simulink model "MRAC_controller"  (R2021b)
settings: Solver=ode113  StartTime=0.0  StopTime=10  RelTol=1e-3
InitFcn:
  | addpath('generated');
  | cst = cellulo_constants();
  | 
  | Td_sens = 0.02;
  | T_ctrl = 0.02;
  | c = cst.c;
  | c_v=cst.c_v;
  | c_F=cst.c_F;
  | c_U = cst.c_U;
  | m = cst.m;
  | d=cst.d;
  | M=mass();
  | 
  | constants = [cst.d;
  |                    cst.c;
  |                    cst.c_F;
  |                    cst.c_U;
  |                    cst.c_v;
  |                    cst.I_drive;
  |                    cst.I_wheel;
  |                    cst.Iz;
  |                    cst.r_mag;
  |                    cst.r_wheel];
  | 
  | rng('default');
  | r = rand(size(constants))/2-0.2;
  | constants = constants + r.*constants;
model workspace (MAT data in the model file):
  Td = 0.1
settings Model: Creator=Hadrien  LastModifiedBy=Hadrien
settings SolverCC: AlgebraicLoopSolver=TrustRegion
settings DebuggingCC: SFMachineParentedDataDiag=warning

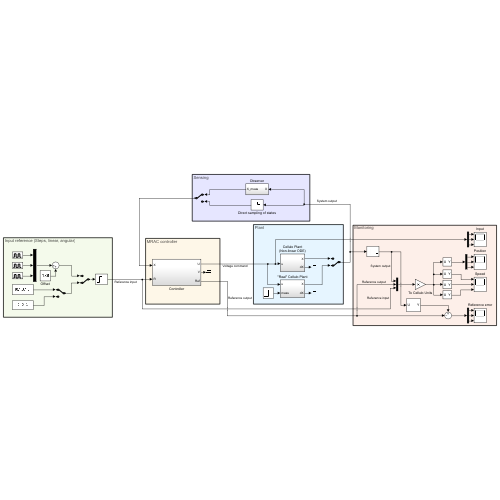
[thumbnail: Simulink's stored preview of the top-level diagram]
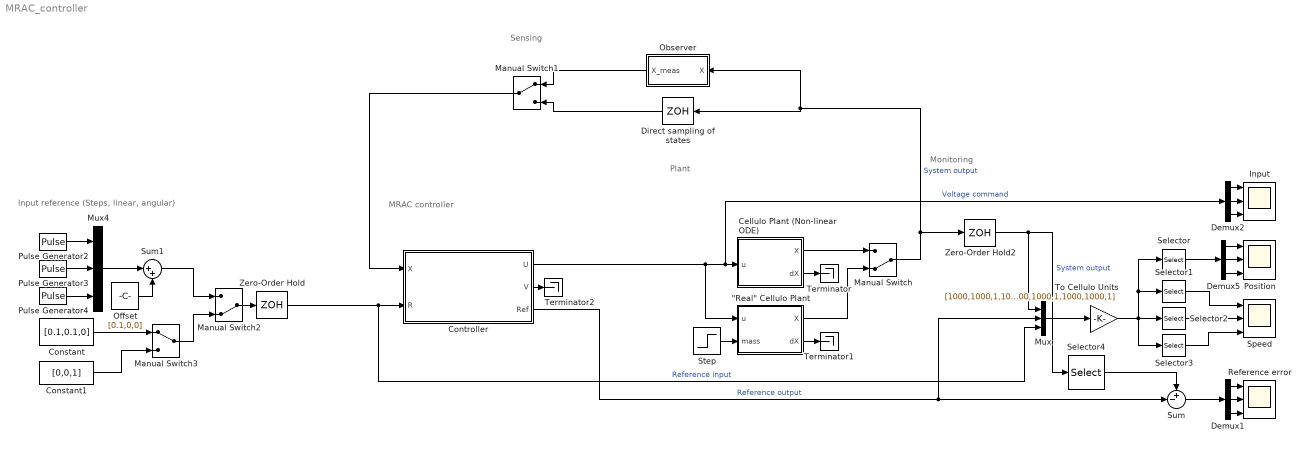
== system MRAC_controller ==
  note: Monitoring
  note: MRAC controller
  note: Plant
  note: Sensing
  note: Input reference (Steps, linear, angular)
  "\"Real\" Cellulo Plant" : Subsystem
  Cellulo Plant (Non-linear ODE) : Subsystem
  Constant : Constant  Value=[0.1,0.1,0]
  Constant1 : Constant  Value=[0,0,1]
  Controller : Subsystem
  Demux1 : Demux  Outputs=3
  Demux2 : Demux  Outputs=3
  Demux5 : Demux  Outputs=3
  Direct sampling of states : ZeroOrderHold  SampleTime=Td_sens
  Input : Scope  NumInputPorts=3
  Manual Switch : ManualSwitch  CurrentSetting=0
  Manual Switch1 : ManualSwitch
  Manual Switch2 : ManualSwitch  CurrentSetting=0
  Manual Switch3 : ManualSwitch
  Mux : Mux  Inputs=3
  Mux4 : Mux  Inputs=3
  Observer : Subsystem
  Offset : Constant  Value=[0.1,0,0]
  Position : Scope  NumInputPorts=3
  Pulse Generator2 : DiscretePulseGenerator  PulseType=Time based  Amplitude=0.1  Period=9  PulseWidth=50  SampleTime=T_ctrl
  Pulse Generator3 : DiscretePulseGenerator  PulseType=Time based  Amplitude=0.1  Period=10  PulseWidth=50  PhaseDelay=2  SampleTime=T_ctrl
  Pulse Generator4 : DiscretePulseGenerator  PulseType=Time based  Period=8  PulseWidth=50  PhaseDelay=1  SampleTime=T_ctrl
  Reference error : Scope  NumInputPorts=3
  Selector : Selector  InputPortWidth=12  IndexOptions=Index vector (dialog)  Indices=[1 2 3]  OutputSizes=1
  Selector1 : Selector  InputPortWidth=12  IndexOptions=Index vector (dialog)  Indices=[4 7 10]  OutputSizes=1
  Selector2 : Selector  InputPortWidth=12  IndexOptions=Index vector (dialog)  Indices=[5 8 11]  OutputSizes=1
  Selector3 : Selector  InputPortWidth=12  IndexOptions=Index vector (dialog)  Indices=[6 9 12]  OutputSizes=1
  Selector4 : Selector  InputPortWidth=6  IndexOptions=Index vector (dialog)  Indices=[4 5 6]  OutputSizes=1
  Speed : Scope  NumInputPorts=3
  Step : Step  Time=0  Before=m  After=10*m  SampleTime=0
  Sum : Sum  Inputs=+-|
  Sum1 : Sum  Inputs=|++
  Terminator : Terminator
  Terminator1 : Terminator
  Terminator2 : Terminator
  To Cellulo Units : Gain  Gain=[1000,1000,1,1000,1000,1,1000,1000,1,1000,1000,1]
  Zero-Order Hold : ZeroOrderHold  SampleTime=T_ctrl
  Zero-Order Hold2 : ZeroOrderHold  SampleTime=T_ctrl
  wires:
  Cellulo Plant (Non-linear ODE)/2(dX) -> Terminator/1
  "\"Real\" Cellulo Plant"/2(dX) -> Terminator1/1
  "\"Real\" Cellulo Plant"/1(X) -> Manual Switch/2
  Cellulo Plant (Non-linear ODE)/1(X) -> Manual Switch/1
  Manual Switch/1 -> Observer/1(X), Direct sampling of states/1, Zero-Order Hold2/1  "System output"
  Observer/1(X_meas) -> Manual Switch1/1
  Direct sampling of states/1 -> Manual Switch1/2
  Controller/1(U) -> Demux2/1, Cellulo Plant (Non-linear ODE)/1(u), "\"Real\" Cellulo Plant"/1(u)  "Voltage command"
  Manual Switch1/1 -> Controller/1(X)
  Step/1 -> "\"Real\" Cellulo Plant"/2(mass)
  Pulse Generator2/1 -> Mux4/1
  Pulse Generator4/1 -> Mux4/3
  Pulse Generator3/1 -> Mux4/2
  Mux/1 -> To Cellulo Units/1
  Selector/1 -> Demux5/1
  Demux5/2 -> Position/2
  Demux5/1 -> Position/1
  Demux5/3 -> Position/3
  Selector1/1 -> Speed/1
  Selector2/1 -> Speed/2
  Selector3/1 -> Speed/3
  To Cellulo Units/1 -> Selector1/1, Selector/1, Selector3/1, Selector2/1
  Zero-Order Hold2/1 -> Selector4/1, Mux/1  "System output"
  Controller/3(Ref) -> Mux/2, Sum/2  "Reference output"
  Demux2/1 -> Input/1
  Demux2/2 -> Input/2
  Demux2/3 -> Input/3
  Controller/2(V) -> Terminator2/1
  Demux1/3 -> Reference error/3
  Demux1/1 -> Reference error/1
  Demux1/2 -> Reference error/2
  Manual Switch2/1 -> Zero-Order Hold/1
  Manual Switch3/1 -> Manual Switch2/2
  Constant/1 -> Manual Switch3/1
  Constant1/1 -> Manual Switch3/2
  Mux4/1 -> Sum1/1
  Sum1/1 -> Manual Switch2/1
  Offset/1 -> Sum1/2
  Zero-Order Hold/1 -> Mux/3, Controller/2(R)  "Reference input"
  Sum/1 -> Demux1/1
  Selector4/1 -> Sum/1

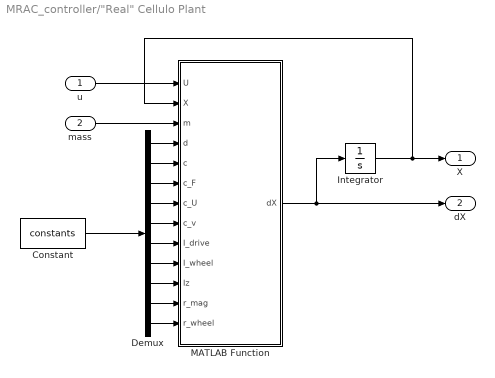
== system MRAC_controller/"Real" Cellulo Plant ==
  u : Inport  PortDimensions=3
  mass : Inport  Port=2
  Constant : Constant  Value=constants
  Demux : Demux  Outputs=10
  Integrator : Integrator
  MATLAB Function : MATLAB Function  TreatAsAtomicUnit=on
  X : Outport  PortDimensions=6
  dX : Outport  Port=2  PortDimensions=6
  wires:
  Integrator/1 -> X/1, MATLAB Function/2(X)
  u/1 -> MATLAB Function/1(U)
  MATLAB Function/1(dX) -> Integrator/1, dX/1
  Demux/1 -> MATLAB Function/4(d)
  Demux/2 -> MATLAB Function/5(c)
  Demux/3 -> MATLAB Function/6(c_F)
  Demux/4 -> MATLAB Function/7(c_U)
  Demux/5 -> MATLAB Function/8(c_v)
  Demux/6 -> MATLAB Function/9(I_drive)
  Demux/7 -> MATLAB Function/10(I_wheel)
  Demux/8 -> MATLAB Function/11(Iz)
  Demux/9 -> MATLAB Function/12(r_mag)
  Demux/10 -> MATLAB Function/13(r_wheel)
  Constant/1 -> Demux/1
  mass/1 -> MATLAB Function/3(m)

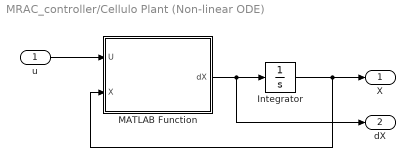
== system MRAC_controller/Cellulo Plant (Non-linear ODE) ==
  u : Inport  PortDimensions=3
  Integrator : Integrator
  MATLAB Function : MATLAB Function  TreatAsAtomicUnit=on
  X : Outport  PortDimensions=6
  dX : Outport  Port=2  PortDimensions=6
  wires:
  u/1 -> MATLAB Function/1(U)
  MATLAB Function/1(dX) -> Integrator/1, dX/1
  Integrator/1 -> MATLAB Function/2(X), X/1

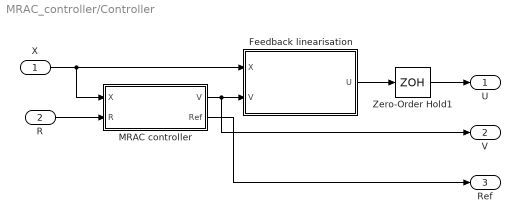
== system MRAC_controller/Controller ==
  X : Inport
  R : Inport  Port=2
  Feedback linearisation : MATLAB Function  TreatAsAtomicUnit=on
  MRAC controller : Subsystem
  Zero-Order Hold1 : ZeroOrderHold  SampleTime=-1
  U : Outport
  V : Outport  Port=2
  Ref : Outport  Port=3
  wires:
  X/1 -> Feedback linearisation/1(X), MRAC controller/1(X)
  R/1 -> MRAC controller/2(R)
  Feedback linearisation/1(U) -> Zero-Order Hold1/1
  MRAC controller/1(V) -> Feedback linearisation/2(V), V/1
  Zero-Order Hold1/1 -> U/1
  MRAC controller/2(Ref) -> Ref/1

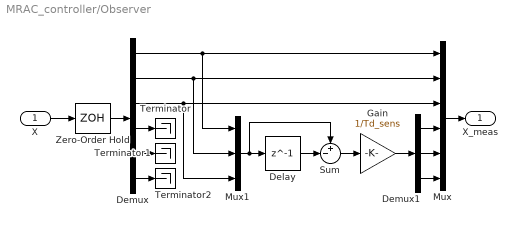
== system MRAC_controller/Observer ==
  X : Inport
  Delay : Delay  DelayLength=1  SampleTime=Td_sens
  Demux : Demux  Outputs=6
  Demux1 : Demux  Outputs=3
  Gain : Gain  Gain=1/Td_sens
  Mux : Mux  Inputs=6
  Mux1 : Mux  Inputs=3
  Sum : Sum  Inputs=+-|
  Terminator : Terminator
  Terminator1 : Terminator
  Terminator2 : Terminator
  Zero-Order Hold : ZeroOrderHold  SampleTime=Td_sens
  X_meas : Outport
  wires:
  X/1 -> Zero-Order Hold/1
  Zero-Order Hold/1 -> Demux/1
  Mux/1 -> X_meas/1
  Demux/1 -> Mux/1, Mux1/1
  Demux/2 -> Mux/2, Mux1/2
  Demux/3 -> Mux/3, Mux1/3
  Demux/4 -> Terminator/1
  Demux/5 -> Terminator1/1
  Demux/6 -> Terminator2/1
  Demux1/1 -> Mux/4
  Demux1/2 -> Mux/5
  Demux1/3 -> Mux/6
  Sum/1 -> Gain/1
  Mux1/1 -> Sum/1, Delay/1
  Delay/1 -> Sum/2
  Gain/1 -> Demux1/1

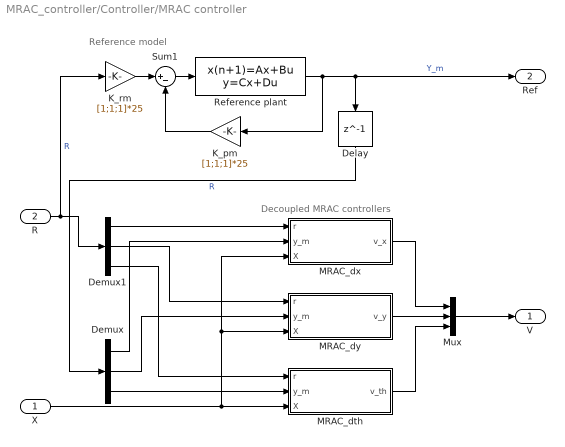
== system MRAC_controller/Controller/MRAC controller ==
  note: Decoupled MRAC controllers
  note: Reference model
  X : Inport
  R : Inport  Port=2
  Delay : Delay  DelayLength=1
  Demux : Demux  Outputs=3
  Demux1 : Demux  Outputs=3
  K_pm : Gain  Gain=[1;1;1]*25
  K_rm : Gain  Gain=[1;1;1]*25
  MRAC_dth : Subsystem
  MRAC_dx : Subsystem
  MRAC_dy : Subsystem
  Mux : Mux  Inputs=3
  Reference plant : DiscreteStateSpace  A=eye(3)  B=T_ctrl*eye(3)  C=eye(3)  D=zeros(3)  SampleTime=-1
  Sum1 : Sum  Inputs=|+-
  V : Outport
  Ref : Outport  Port=2
  wires:
  K_pm/1 -> Sum1/2
  K_rm/1 -> Sum1/1
  Sum1/1 -> Reference plant/1
  Reference plant/1 -> Ref/1, Delay/1, K_pm/1  "Y_m"
  Demux/1 -> MRAC_dx/2(y_m)
  Demux1/1 -> MRAC_dx/1(r)
  X/1 -> MRAC_dy/3(X), MRAC_dx/3(X), MRAC_dth/3(X)
  MRAC_dx/1(v_x) -> Mux/1
  Demux1/2 -> MRAC_dy/1(r)
  Demux1/3 -> MRAC_dth/1(r)
  Demux/2 -> MRAC_dy/2(y_m)
  Demux/3 -> MRAC_dth/2(y_m)
  MRAC_dy/1(v_y) -> Mux/2
  MRAC_dth/1(v_th) -> Mux/3
  Mux/1 -> V/1
  R/1 -> K_rm/1, Demux1/1  "R"
  Delay/1 -> Demux/1  "R"

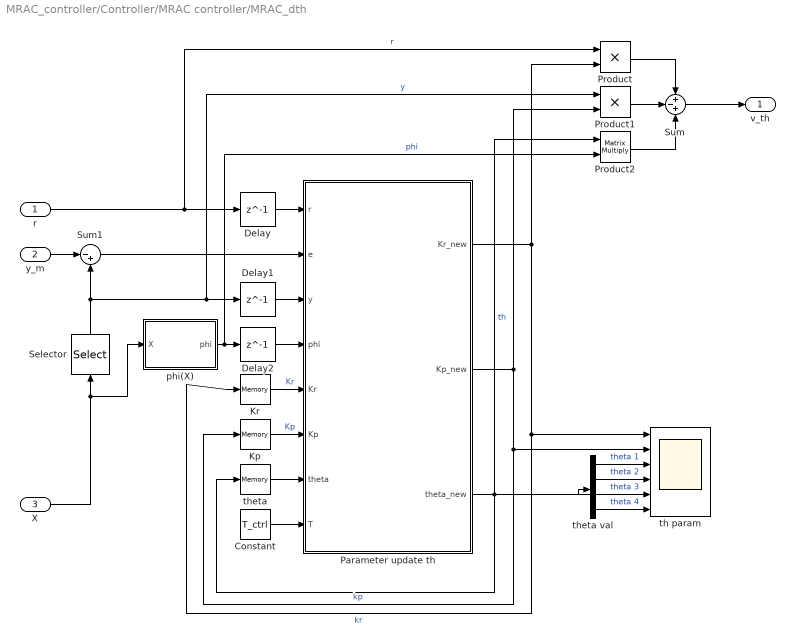
== system MRAC_controller/Controller/MRAC controller/MRAC_dth ==
  r : Inport
  y_m : Inport  Port=2
  X : Inport  Port=3
  Constant : Constant  Value=T_ctrl
  Delay : Delay  DelayLength=1
  Delay1 : Delay  DelayLength=1
  Delay2 : Delay  DelayLength=1
  Kp : Memory  InitialCondition=118  InheritSampleTime=on
  Kr : Memory  InitialCondition=119  InheritSampleTime=on
  Parameter update th : MATLAB Function  TreatAsAtomicUnit=on
  Product : Product
  Product1 : Product
  Product2 : Product  Multiplication=Matrix(*)
  Selector : Selector  InputPortWidth=6  IndexOptions=Index vector (dialog)  Indices=6  OutputSizes=1
  Sum : Sum  Inputs=+-+
  Sum1 : Sum  Inputs=|-+
  phi(X) : MATLAB Function  TreatAsAtomicUnit=on
  th param : Scope  NumInputPorts=6
  theta : Memory  InitialCondition=[368.75,11.94,11.94,11.94]  InheritSampleTime=on
  theta val : Demux
  v_th : Outport
  wires:
  X/1 -> phi(X)/1(X), Selector/1
  Sum/1 -> v_th/1
  r/1 -> Product/1, Delay/1  "r"
  Selector/1 -> Product1/1, Delay1/1, Sum1/2  "y"
  y_m/1 -> Sum1/1
  theta val/1 -> th param/3  "theta 1"
  theta val/3 -> th param/5  "theta 3"
  theta val/2 -> th param/4  "theta 2"
  theta val/4 -> th param/6  "theta 4"
  Delay/1 -> Parameter update th/1(r)
  Sum1/1 -> Parameter update th/2(e)
  Delay1/1 -> Parameter update th/3(y)
  Delay2/1 -> Parameter update th/4(phi)
  Kr/1 -> Parameter update th/5(Kr)  "Kr"
  Kp/1 -> Parameter update th/6(Kp)  "Kp"
  theta/1 -> Parameter update th/7(theta)
  Constant/1 -> Parameter update th/8(T)
  phi(X)/1(phi) -> Product2/2, Delay2/1  "phi"
  Parameter update th/3(theta_new) -> Product2/1, theta/1, theta val/1  "th"
  Parameter update th/2(Kp_new) -> Product1/2, th param/2, Kp/1  "kp"
  Parameter update th/1(Kr_new) -> Product/2, th param/1, Kr/1  "kr"
  Product/1 -> Sum/1
  Product1/1 -> Sum/2
  Product2/1 -> Sum/3

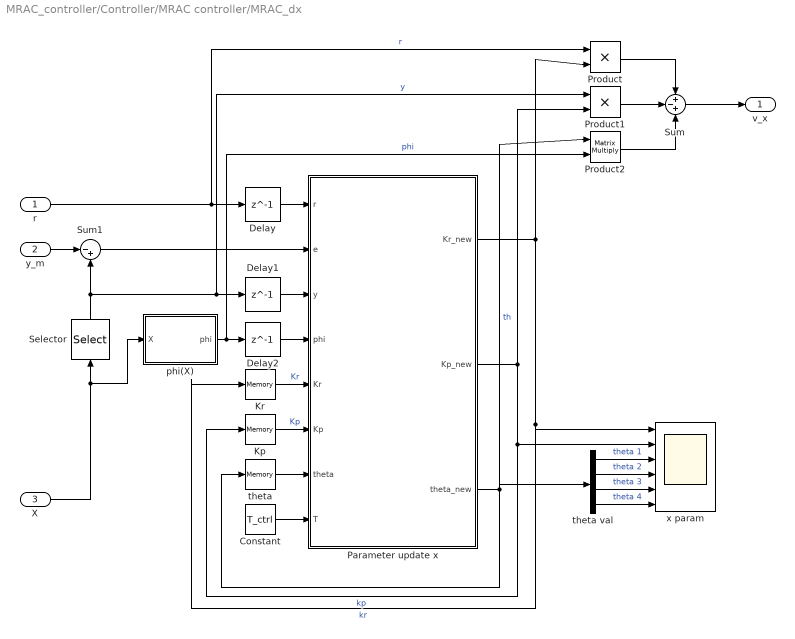
== system MRAC_controller/Controller/MRAC controller/MRAC_dx ==
  r : Inport
  y_m : Inport  Port=2
  X : Inport  Port=3
  Constant : Constant  Value=T_ctrl
  Delay : Delay  DelayLength=1
  Delay1 : Delay  DelayLength=1
  Delay2 : Delay  DelayLength=1
  Kp : Memory  InitialCondition=48.5  InheritSampleTime=on
  Kr : Memory  InitialCondition=46.5  InheritSampleTime=on
  Parameter update x : MATLAB Function  TreatAsAtomicUnit=on
  Product : Product
  Product1 : Product
  Product2 : Product  Multiplication=Matrix(*)
  Selector : Selector  InputPortWidth=6  IndexOptions=Index vector (dialog)  Indices=4  OutputSizes=1
  Sum : Sum  Inputs=+-+
  Sum1 : Sum  Inputs=|-+
  phi(X) : MATLAB Function  TreatAsAtomicUnit=on
  theta : Memory  InitialCondition=[114.25,0.185,0.185,0.185]  InheritSampleTime=on
  theta val : Demux
  x param : Scope  NumInputPorts=6
  v_x : Outport
  wires:
  Sum/1 -> v_x/1
  theta val/4 -> x param/6  "theta 4"
  theta val/2 -> x param/4  "theta 2"
  theta val/3 -> x param/5  "theta 3"
  theta val/1 -> x param/3  "theta 1"
  X/1 -> phi(X)/1(X), Selector/1
  Selector/1 -> Sum1/2, Product1/1, Delay1/1  "y"
  y_m/1 -> Sum1/1
  r/1 -> Product/1, Delay/1  "r"
  Delay/1 -> Parameter update x/1(r)
  Sum1/1 -> Parameter update x/2(e)
  Delay1/1 -> Parameter update x/3(y)
  phi(X)/1(phi) -> Product2/2, Delay2/1  "phi"
  Delay2/1 -> Parameter update x/4(phi)
  Kr/1 -> Parameter update x/5(Kr)  "Kr"
  Kp/1 -> Parameter update x/6(Kp)  "Kp"
  theta/1 -> Parameter update x/7(theta)
  Constant/1 -> Parameter update x/8(T)
  Parameter update x/3(theta_new) -> Product2/1, theta/1, theta val/1  "th"
  Parameter update x/2(Kp_new) -> Product1/2, x param/2, Kp/1  "kp"
  Parameter update x/1(Kr_new) -> x param/1, Kr/1, Product/2  "kr"
  Product1/1 -> Sum/2
  Product/1 -> Sum/1
  Product2/1 -> Sum/3

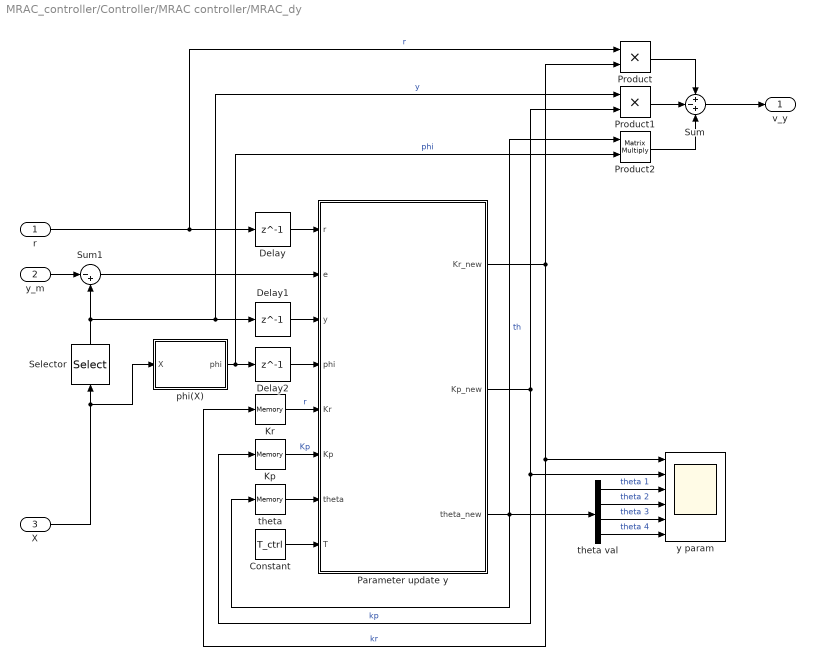
== system MRAC_controller/Controller/MRAC controller/MRAC_dy ==
  r : Inport
  y_m : Inport  Port=2
  X : Inport  Port=3
  Constant : Constant  Value=T_ctrl
  Delay : Delay  DelayLength=1
  Delay1 : Delay  DelayLength=1
  Delay2 : Delay  DelayLength=1
  Kp : Memory  InitialCondition=48.5  InheritSampleTime=on
  Kr : Memory  InitialCondition=46.5  InheritSampleTime=on
  Parameter update y : MATLAB Function  TreatAsAtomicUnit=on
  Product : Product
  Product1 : Product
  Product2 : Product  Multiplication=Matrix(*)
  Selector : Selector  InputPortWidth=6  IndexOptions=Index vector (dialog)  Indices=5  OutputSizes=1
  Sum : Sum  Inputs=+-+
  Sum1 : Sum  Inputs=|-+
  phi(X) : MATLAB Function  TreatAsAtomicUnit=on
  theta : Memory  InitialCondition=[114.2,0.205,0.205,0.205]  InheritSampleTime=on
  theta val : Demux
  y param : Scope  NumInputPorts=6
  v_y : Outport
  wires:
  X/1 -> phi(X)/1(X), Selector/1
  Sum/1 -> v_y/1
  Selector/1 -> Product1/1, Delay1/1, Sum1/2  "y"
  y_m/1 -> Sum1/1
  theta val/4 -> y param/6  "theta 4"
  theta val/2 -> y param/4  "theta 2"
  theta val/3 -> y param/5  "theta 3"
  theta val/1 -> y param/3  "theta 1"
  r/1 -> Product/1, Delay/1  "r"
  Sum1/1 -> Parameter update y/2(e)
  Delay/1 -> Parameter update y/1(r)
  Delay1/1 -> Parameter update y/3(y)
  Delay2/1 -> Parameter update y/4(phi)
  phi(X)/1(phi) -> Product2/2, Delay2/1  "phi"
  Kr/1 -> Parameter update y/5(Kr)  "r"
  Kp/1 -> Parameter update y/6(Kp)  "Kp"
  theta/1 -> Parameter update y/7(theta)
  Constant/1 -> Parameter update y/8(T)
  Parameter update y/3(theta_new) -> theta val/1, Product2/1, theta/1  "th"
  Parameter update y/2(Kp_new) -> Product1/2, y param/2, Kp/1  "kp"
  Parameter update y/1(Kr_new) -> Product/2, y param/1, Kr/1  "kr"
  Product/1 -> Sum/1
  Product1/1 -> Sum/2
  Product2/1 -> Sum/3

== matlab function MRAC_controller/Controller/MRAC controller/MRAC_dy/phi(X) ==
  data: X input; phi output
function phi = phi(X)

th=X(3);
dx=X(4);
dy=X(5);
dth=X(6);

c1=sign(-cos(th)*dx-sin(th)*dy+0.028*dth);
c2=sign(cos(th-pi/3)*dx-cos(th+pi/6)*dy+0.028*dth);
c3=sign(cos(th+pi/3)*dx+sin(th+pi/3)*dy+0.028*dth);

phi = [dy;-sin(th)*c1;-cos(th+pi/6)*c2;sin(th+pi/3)*c3];

== matlab function MRAC_controller/Controller/MRAC controller/MRAC_dth/Parameter update th ==
  data: Kr_new output; r input; e input; y input; Kp_new output; phi input; Kr input; theta_new output; Kp input; theta input; T input
function [Kr_new,Kp_new,theta_new] = update(r,e,y,phi,Kr,Kp,theta,T)

theta_v=reshape(theta,[1,4]);
dtheta=zeros(1,4);

gamma_p = 1000;
gamma_r = 1000;
Gamma = 100*diag([1,1,1,1]);

dKp = gamma_p*y*e;
dKr = -gamma_r*r*e;
dtheta = -(Gamma*phi*e)';

Kp_new = Kp + T*dKp;
Kr_new = Kr + T*dKr;
theta_new = theta_v + T*dtheta;

== matlab function MRAC_controller/Controller/MRAC controller/MRAC_dth/phi(X) ==
  data: X input; phi output
function phi = phi(X)

th=X(3);
dx=X(4);
dy=X(5);
dth=X(6);

c1=sign(-cos(th)*dx-sin(th)*dy+0.028*dth);
c2=sign(cos(th-pi/3)*dx-cos(th+pi/6)*dy+0.028*dth);
c3=sign(cos(th+pi/3)*dx+sin(th+pi/3)*dy+0.028*dth);

phi = [dth;c1;c2;c3];

== matlab function MRAC_controller/Controller/Feedback linearisation ==
  data: X input; V input; U output
function U = Inverse_dynamics(X,V)

th = X(3);
w1 = V(1);
w2 = V(2);
w3 = V(3);

M = mass();
Q = input_forces(th);

U = Q\(M*[w1;w2;w3]);

== matlab function MRAC_controller/Cellulo Plant (Non-linear ODE)/MATLAB Function ==
  data: U input; X input; dX output
function dX = Cellulo_ODE(U,X)

x = X(1);
y = X(2);
th = X(3);
dx = X(4);
dy = X(5);
dth = X(6);
u1 = U(1);
u2 = U(2);
u3 = U(3);

M = mass();
C = coriolis();
G = gravity();
D = friction(dth,dx,dy,th);
Q = input_forces(th);
dq = reshape(X(4:6),3,1);
ddq = M\(-C*dq - G - D + Q*[u1;u2;u3]);
dX = [dq;ddq];

== matlab function MRAC_controller/"Real" Cellulo Plant/MATLAB Function ==
  data: U input; X input; m input; d input; c input; c_F input; c_U input; c_v input; dX output; I_drive input; I_wheel input; Iz input; r_mag input; r_wheel input
function dX = Cellulo_ODE(U,X,m,d,c,c_F,c_U,c_v,I_drive,I_wheel,Iz,r_mag,r_wheel)

x = X(1);
y = X(2);
th = X(3);
dx = X(4);
dy = X(5);
dth = X(6);
u1 = U(1);
u2 = U(2);
u3 = U(3);

M = mass_symbolic(I_drive,I_wheel,Iz,d,m,r_mag,r_wheel);
C = coriolis_symbolic();
G = gravity_symbolic();
D = friction_symbolic(c,c_F,c_v,d,dth,dx,dy,th);
Q = input_forces_symbolic(c_F,c_U,d,th);
dq = reshape(X(4:6),3,1);
ddq = M\(-C*dq - G - D + Q*[u1;u2;u3]);
dX = [dq;ddq];

== matlab function MRAC_controller/Controller/MRAC controller/MRAC_dx/phi(X) ==
  data: X input; phi output
function phi = phi(X)

th=X(3);
dx=X(4);
dy=X(5);
dth=X(6);

c1=sign(-cos(th)*dx    -sin(th)*dy     +0.028*dth);
c2=sign(cos(th-pi/3)*dx-cos(th+pi/6)*dy+0.028*dth);
c3=sign(cos(th+pi/3)*dx+sin(th+pi/3)*dy+0.028*dth);

phi = [dx;-cos(th)*c1;cos(th-pi/3)*c2;cos(th+pi/3)*c3];

== matlab function MRAC_controller/Controller/MRAC controller/MRAC_dx/Parameter update x ==
  data: Kr_new output; r input; e input; y input; Kp_new output; phi input; Kr input; theta_new output; Kp input; theta input; T input
function [Kr_new,Kp_new,theta_new] = update(r,e,y,phi,Kr,Kp,theta,T)

theta_v=reshape(theta,[1,4]);
dtheta=zeros(1,4);

gamma_p = 10000;
gamma_r = 10000;
Gamma = 10*diag([100,1,1,1]);

dKp = gamma_p*y*e;
dKr = -gamma_r*r*e;
dtheta = -(Gamma*phi*e)';

Kp_new = Kp + T*dKp;
Kr_new = Kr + T*dKr;
theta_new = theta_v + T*dtheta;

== matlab function MRAC_controller/Controller/MRAC controller/MRAC_dy/Parameter update y ==
  data: Kr_new output; r input; e input; y input; Kp_new output; phi input; Kr input; theta_new output; Kp input; theta input; T input
function [Kr_new,Kp_new,theta_new] = update(r,e,y,phi,Kr,Kp,theta,T)

theta_v=reshape(theta,[1,4]);
dtheta=zeros(1,4);

gamma_p = 10000;
gamma_r = 10000;
Gamma = 10*diag([100,1,1,1]);

dKp = gamma_p*y*e;
dKr = -gamma_r*r*e;
dtheta = -(Gamma*phi*e)';

Kp_new = Kp + T*dKp;
Kr_new = Kr + T*dKr;
theta_new = theta_v + T*dtheta;
